simulink model "gm_calk"  (R2022a)
settings: Solver=VariableStepAuto  StartTime=0.0  StopTime=10.0  RelTol=1e-3
settings Model: Creator=Vova  LastModifiedBy=Vova
settings OptimizationCC: BlockReduction=off  ConditionallyExecuteInputs=off
settings DebuggingCC: InheritedTsInSrcMsg=none

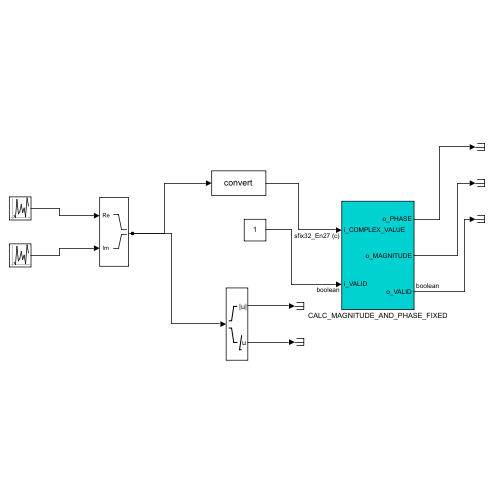
[thumbnail: Simulink's stored preview of the top-level diagram]
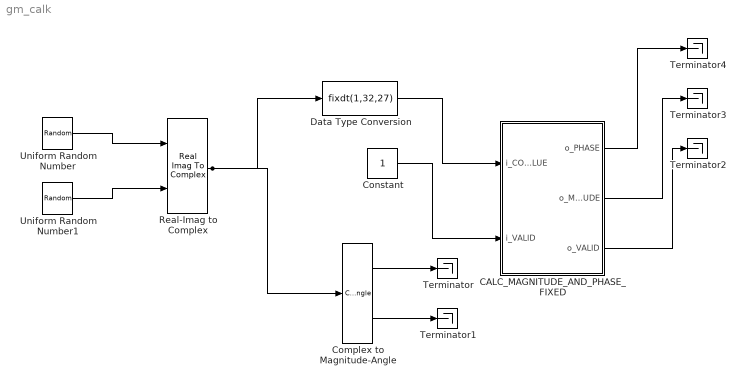
== system gm_calk ==
  CALC_MAGNITUDE_AND_PHASE_FIXED : Subsystem
  Complex to Magnitude-Angle : ComplexToMagnitudeAngle
  Constant : Constant  OutDataTypeStr=boolean  SampleTime=1
  Data Type Conversion : DataTypeConversion  OutDataTypeStr=fixdt(1,32,27)  RndMeth=Round  SaturateOnIntegerOverflow=off
  Real-Imag to Complex : RealImagToComplex
  Terminator{,1..4} (5 alike) : Terminator
  Uniform Random Number : UniformRandomNumber  Minimum=0  Maximum=31.9999999254941940308  Seed=5  SampleTime=1
  Uniform Random Number1 : UniformRandomNumber  Minimum=0  Maximum=31.9999999254941940308  Seed=6  SampleTime=1
  wires:
  CALC_MAGNITUDE_AND_PHASE_FIXED/1(o_PHASE) -> Terminator4/1
  Uniform Random Number1/1 -> Real-Imag to Complex/2
  Data Type Conversion/1 -> CALC_MAGNITUDE_AND_PHASE_FIXED/1(i_COMPLEX_VALUE)
  CALC_MAGNITUDE_AND_PHASE_FIXED/3(o_VALID) -> Terminator2/1
  Constant/1 -> CALC_MAGNITUDE_AND_PHASE_FIXED/2(i_VALID)
  Uniform Random Number/1 -> Real-Imag to Complex/1
  Complex to Magnitude-Angle/2 -> Terminator1/1
  CALC_MAGNITUDE_AND_PHASE_FIXED/2(o_MAGNITUDE) -> Terminator3/1
  Complex to Magnitude-Angle/1 -> Terminator/1
  Real-Imag to Complex/1 -> Complex to Magnitude-Angle/1, Data Type Conversion/1

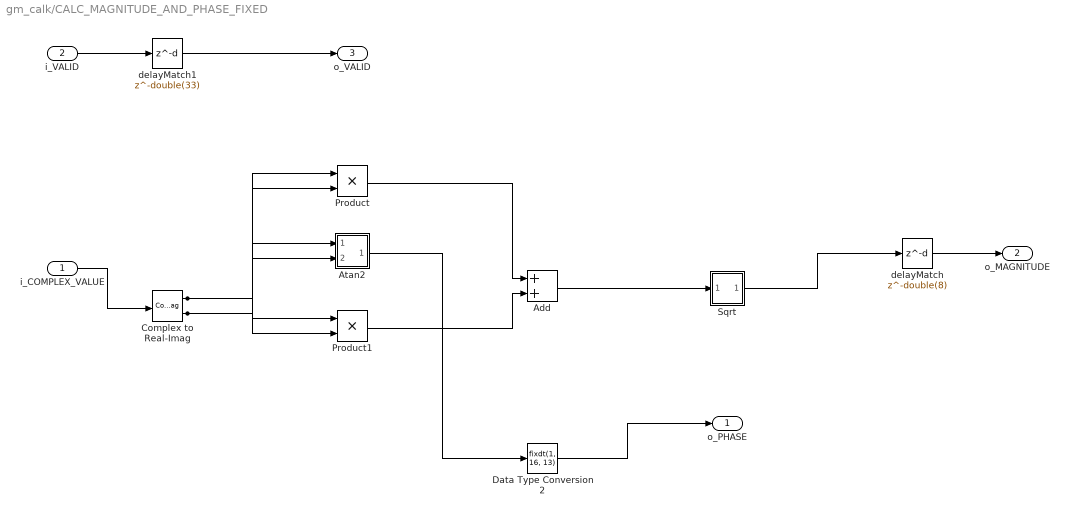
== system gm_calk/CALC_MAGNITUDE_AND_PHASE_FIXED ==
  i_COMPLEX_VALUE : Inport  OutDataTypeStr=fixdt(1, 32, 27)  PortDimensions=1  SampleTime=1
      settings: SignalType=complex
  i_VALID : Inport  Port=2  OutDataTypeStr=boolean  PortDimensions=1  SampleTime=1
  Add : Sum  AccumDataTypeStr=fixdt(1, 65, 54)  OutDataTypeStr=fixdt(0, 65, 55)  SampleTime=1
  Atan2 : Subsystem
  Complex to Real-Imag : ComplexToRealImag  SampleTime=1
  Data Type Conversion2 : DataTypeConversion  OutDataTypeStr=fixdt(1, 16, 13)  SampleTime=1  SaturateOnIntegerOverflow=off  RndMeth=Floor
  Product : Product  Inputs=**  OutDataTypeStr=fixdt(1, 64, 54)  SaturateOnIntegerOverflow=on  SampleTime=1
  Product1 : Product  Inputs=**  OutDataTypeStr=fixdt(1, 64, 54)  SampleTime=1
  Sqrt : Subsystem
  delayMatch : Delay  DelayLength=double(8)  InitialCondition=0  SampleTime=1
  delayMatch1 : Delay  DelayLength=double(33)  InitialCondition=0  SampleTime=1
  o_PHASE : Outport  SampleTime=1
  o_MAGNITUDE : Outport  Port=2  SampleTime=1
  o_VALID : Outport  Port=3  OutDataTypeStr=boolean  SampleTime=1
  wires:
  i_COMPLEX_VALUE/1 -> Complex to Real-Imag/1
  delayMatch1/1 -> o_VALID/1
  Add/1 -> Sqrt/1(In1)
  Atan2/1(Out1) -> Data Type Conversion2/1
  Complex to Real-Imag/1 -> Product/2, Product/1, Atan2/2(In2)
  Complex to Real-Imag/2 -> Product1/2, Product1/1, Atan2/1(In1)
  Data Type Conversion2/1 -> o_PHASE/1
  Product/1 -> Add/1
  Product1/1 -> Add/2
  delayMatch/1 -> o_MAGNITUDE/1
  Sqrt/1(Out1) -> delayMatch/1
  i_VALID/1 -> delayMatch1/1

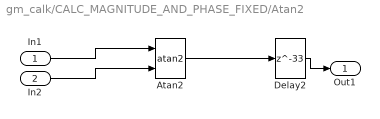
== system gm_calk/CALC_MAGNITUDE_AND_PHASE_FIXED/Atan2 ==
  In1 : Inport
  In2 : Inport  Port=2
  Atan2 : Trigonometry  Operator=atan2  ApproximationMethod=CORDIC  NumberOfIterations=30
  Delay2 : Delay  DelayLength=33
  Out1 : Outport
  wires:
  In1/1 -> Atan2/1
  In2/1 -> Atan2/2
  Atan2/1 -> Delay2/1
  Delay2/1 -> Out1/1

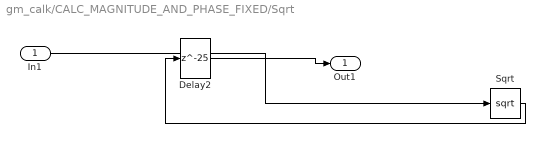
== system gm_calk/CALC_MAGNITUDE_AND_PHASE_FIXED/Sqrt ==
  In1 : Inport
  Delay2 : Delay  DelayLength=25
  Sqrt : Sqrt  OutDataTypeStr=fixdt(1,33,18)
  Out1 : Outport
  wires:
  In1/1 -> Sqrt/1
  Sqrt/1 -> Delay2/1
  Delay2/1 -> Out1/1
